simulink model "Frequency_Recovery_Closed_Loop"  (Simulink 8.6)
settings: Solver=FixedStepDiscrete  StartTime=0  StopTime=inf  RelTol=1e-3
InitFcn:
  | % Trainingssequenz
  | trainseq=1/sqrt(2) * ((2*randi([0 1],32,1)-1) + 1i * (2*randi([0 1],32,1)-1));
undefined symbols (not defined in the file): gcbh, rcfiltgaincompat
libraries: commchan3 x1, dspsrcs4 x1, simulink x1, commdigbbndpm3 x1, commrandsrc2 x1, commfilt2 x1
settings Model: Creator=schwall  LastModifiedBy=wunsch
settings DataIOCC: SaveOutput=off  SignalLogging=off  SaveTime=off
settings DebuggingCC: InheritedTsInSrcMsg=none  FcnCallInpInsideContextMsg=UseLocalSettings
settings SFSimCC: SimParseCustomCode=off

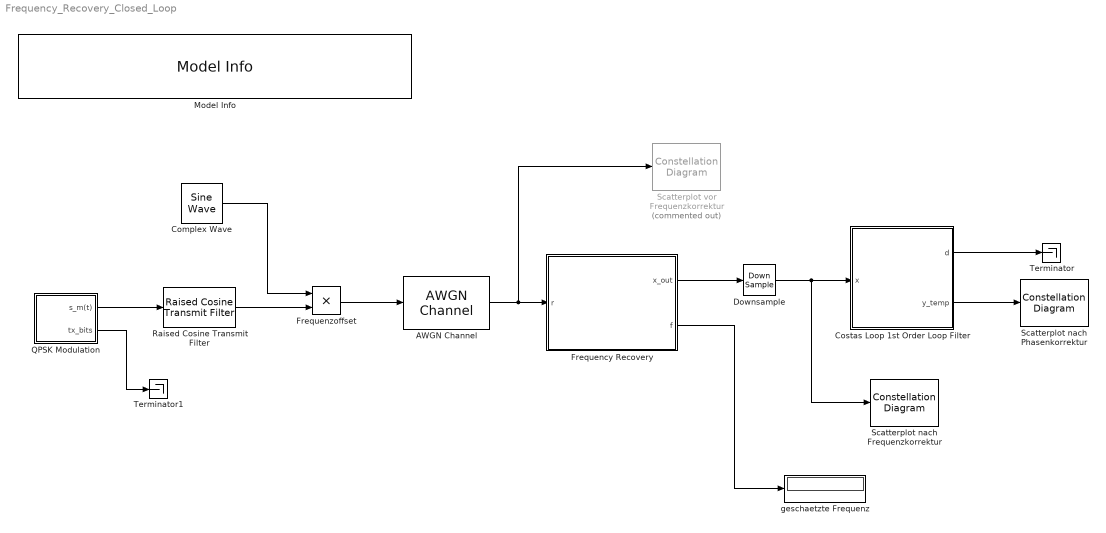
== system Frequency_Recovery_Closed_Loop ==
  AWGN Channel : commchan3/AWGN Channel  InputProcessing=Columns as channels (frame based)  seed=67  noiseMode="Signal to noise ratio  (Es/No)"  EbNodB=12  EsNodB=30  SNRdB=10  bitsPerSym=2  Ps=1/8  Tsym=0.128/128/8  variance=1
  Complex Wave : dspsrcs4/Sine Wave  Amplitude=1  Frequency=0  Phase=0  SampleMode=Discrete  OutComplex=Complex  CompMethod=Trigonometric fcn  TableSize=Speed  SampleTime=0.128/128/8  SamplesPerFrame=1024  ResetState=Restart at time zero  OutputFrames=on  dataType=double  wordLen=16  udDataType=sfix(16)  fracBitsMode=Best precision  numFracBits=15  OutDataTypeStr=double  LastOutDataTypeStr=double
  Costas Loop 1st Order Loop Filter : MATLAB Function  TreatAsAtomicUnit=on
  Downsample : DownSample
  Frequency Recovery : MATLAB Function  TreatAsAtomicUnit=on
  Frequenzoffset : Product  RndMeth=Zero
  Model Info : simulink/Model-Wide Utilities/Model Info  BlockCM=None  Frame=on  DisplayStringWithTags=|  HorizontalTextAlignment=Left  LeftAlignmentValue=0.02  SourceBlockDiagram=Frequency_Recovery_Closed_Loop  TagMaxNumber=20
      | Demo Frequency Recovery Closed Loop
      | Vorlesung Nachrichtentechnik II
      | Institut fuer Nachrichtentechnik (CEL)
  QPSK Modulation : Subsystem
  Raised Cosine Transmit Filter : commfilt2/Raised Cosine Transmit Filter  filtType=Square root  filtSpan=2*(3)  currentFiltSpan=2*(3)  D=3  R=0.35  sampMode=Mute  saveAsFlag=0  N=8  framing=Enforce single-rate processing  InputProcessing=Columns as channels (frame based)  checkGain=Normalized  filterGain=rcfiltgaincompat(gcbh)  checkCoeff=off  variableName=rcTxFilt  launchFVT=off  roundingMode=Floor  overflowMode=off
  Scatterplot nach Frequenzkorrektur : ConstellationDiagram  Tag=ScatterPlot
  Scatterplot nach Phasenkorrektur : ConstellationDiagram  Tag=ScatterPlot
  Scatterplot vor Frequenzkorrektur : ConstellationDiagram  Tag=ScatterPlot  Commented=on
  Terminator : Terminator
  Terminator1 : Terminator
  geschaetzte Frequenz : Display
  wires:
  QPSK Modulation/1(s_m(t)) -> Raised Cosine Transmit Filter/1
  Frequenzoffset/1 -> AWGN Channel/1
  Complex Wave/1 -> Frequenzoffset/1
  Raised Cosine Transmit Filter/1 -> Frequenzoffset/2
  AWGN Channel/1 -> Scatterplot vor Frequenzkorrektur/1, Frequency Recovery/1(r)
  Frequency Recovery/1(x_out) -> Downsample/1
  Frequency Recovery/2(f) -> geschaetzte Frequenz/1
  Costas Loop 1st Order Loop Filter/2(y_temp) -> Scatterplot nach Phasenkorrektur/1
  Downsample/1 -> Scatterplot nach Frequenzkorrektur/1, Costas Loop 1st Order Loop Filter/1(x)
  Costas Loop 1st Order Loop Filter/1(d) -> Terminator/1
  QPSK Modulation/2(tx_bits) -> Terminator1/1

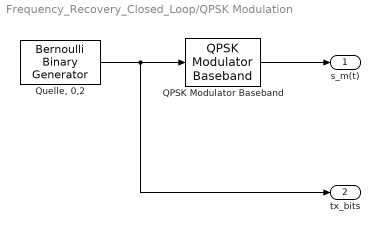
== system Frequency_Recovery_Closed_Loop/QPSK Modulation ==
  QPSK Modulator Baseband : commdigbbndpm3/QPSK Modulator Baseband  InType=Bit  Enc=Gray  Ph=pi/4  outDtype=double  outWordLen=16  outUDDataType=sfix(16)  outFracLenMode=Best precision  outFracLen=15
  "Quelle, 0,2" : commrandsrc2/Bernoulli Binary Generator  P=0.5  seed=61  Ts=1/1000/2  frameBased=on  sampPerFrame=256  orient=off  outDataType=double
  s_m(t) : Outport
  tx_bits : Outport  Port=2
  wires:
  "Quelle, 0,2"/1 -> QPSK Modulator Baseband/1, tx_bits/1
  QPSK Modulator Baseband/1 -> s_m(t)/1

== matlab function Frequency Recovery ==
  data: x_out output double; r input double; f output double
function [x_out,f]  = recovery(r)
%#codegen

%%%%%%%%%%%%%%%%%%%%%%%%%%%%%%%%%%%%%%%%%%%%%%%%%%%%%%%%%%%%%%%%%%%%%%%%%%%
% Initalisierung
%%%%%%%%%%%%%%%%%%%%%%%%%%%%%%%%%%%%%%%%%%%%%%%%%%%%%%%%%%%%%%%%%%%%%%%%%%%

% Impulsantwort Matched Filter
g_mf = [-0.00899923276653125,-0.00862010031857740,-0.00522380865789863,0.00100721609395230,0.00905626800252464,0.0171605778586790,0.0231027321668600,0.0246690244769097,0.0201947243108860,0.00908564037698491,-0.00780385491973082,-0.0280398387740470,-0.0477877316963890,-0.0623056364195982,-0.0666918594078338,-0.0567682669013122,-0.0299425306660226,0.0141173785993224,0.0731400166589809,0.142329093949593,0.214880423378019,0.282872674533704,0.338395135492808,0.374726714857473,0.387365059213122,0.374726714857473,0.338395135492808,0.282872674533704,0.214880423378019,0.142329093949593,0.0731400166589809,0.0141173785993224,-0.0299425306660226,-0.0567682669013122,-0.0666918594078338,-0.0623056364195982,-0.0477877316963890,-0.0280398387740470,-0.00780385491973082,0.00908564037698491,0.0201947243108860,0.0246690244769097,0.0231027321668600,0.0171605778586790,0.00905626800252464,0.00100721609395230,-0.00522380865789863,-0.00862010031857740,-0.00899923276653125];
% Derivative Matched Filter
T = 1;
k = ceil(-length(g_mf)/2):floor(length(g_mf)/2);
g_dmf = 2*pi*T*k.*g_mf;

% Ausgabe initialisieren
x_out = complex(zeros(length(r)/4,1));
f = 0;

% Schrittweite
gamma = 0.01;

% temp. Variable: Speicherinhalt x-Zweig
persistent x_buf
if isempty(x_buf)
    x_buf = complex(zeros(length(g_mf)-1,1));
end

persistent x_1
if isempty(x_1)
    x_1 = complex(0);
end

% temp. Variable: Speicherinhalt y-Zweig
persistent y_buf
if isempty(y_buf)
    y_buf = complex(zeros(length(g_dmf)-1,1));
end

persistent y_1
if isempty(y_1)
    y_1 = complex(0);
end

% Frequenz
persistent nu
if isempty(nu)
    nu = 0;
end

% Phaseninkrement
persistent phi
if isempty(phi)
    phi = 0;
end

% temp. Zaehlervariable
cnt=1;

%%%%%%%%%%%%%%%%%%%%%%%%%%%%%%%%%%%%%%%%%%%%%%%%%%%%%%%%%%%%%%%%%%%%%%%%%%%
% Phasenkorrektur
%%%%%%%%%%%%%%%%%%%%%%%%%%%%%%%%%%%%%%%%%%%%%%%%%%%%%%%%%%%%%%%%%%%%%%%%%%%

for ii=1:length(r)
    
    % Korrektur des Eingangswertes
    r(ii) = r(ii) * exp(1i*(-phi));
    
    % neues Phaseninkrement berechnen
    phi = phi + 2*pi*nu/8000;
    
    % Filteroperationen, MF+DMF
    [x,x_buf] = filter(g_mf, 1,r(ii),x_buf);
    [y,y_buf] = filter(g_dmf,1,r(ii),y_buf);
    
      
    % Downsample by 8
    if (mod(ii,8) == 1)
        
        % Fehler berechnen
        e = 0.5*imag(x_1*conj(y_1)) + 0.5*imag(x*conj(y)); 
        
        % Frequenzoffset berechnen
        nu= nu + gamma*e;     
        
        % nur zur Visualisierung
        f=f+nu;
    end
    
    % Downsample by 4
    if (mod(ii,4) == 1)
        
        x_1 = x;
        y_1 = y;
        
        % Ausgabe, Faktor 2 ueberabgetastet!
        x_out(cnt) = x;
        cnt=cnt+1;
    end    
   
end

% nur zur Visualisierung
f=f/length(r)*8;

== matlab function Costas Loop 1st Order Loop Filter ==
  data: x input double; d output double; y_temp output double
function [d,y_temp] = recovery(x)
%#codegen

%%%%%%%%%%%%%%%%%%%%%%%%%%%%%%%%%%%%%%%%%%%%%%%%%%%%%%%%%%%%%%%%%%%%%%%%%%%
% Initalisierung
%%%%%%%%%%%%%%%%%%%%%%%%%%%%%%%%%%%%%%%%%%%%%%%%%%%%%%%%%%%%%%%%%%%%%%%%%%%

gamma       = 0.5;                          % Schrittweite

persistent phi
if isempty(phi)
    phi = 0;
end

d = complex(zeros(length(x),1));            % Ausgabevektor

y_temp=complex(zeros(length(x),1));         % nur fuer Visualisierungszwecke

%%%%%%%%%%%%%%%%%%%%%%%%%%%%%%%%%%%%%%%%%%%%%%%%%%%%%%%%%%%%%%%%%%%%%%%%%%%
% Phasenkorrektur
%%%%%%%%%%%%%%%%%%%%%%%%%%%%%%%%%%%%%%%%%%%%%%%%%%%%%%%%%%%%%%%%%%%%%%%%%%%

for ii=1:length(x)
    
    
    % Korrektur des Eingangswertes
    y = x(ii) * exp(1i*(-phi));
    
    % nur fuer Visualisierungszwecke
    y_temp(ii) = y;
    
    % Detektor
    d(ii) = detector(y);
    
      
    % Bestimmung des Phasenkorrekturwertes
    phi = phi + gamma * imag( conj(d(ii)) * y );
    
    
end

end


%%%%%%%%%%%%%%%%%%%%%%%%%%%%%%%%%%%%%%%%%%%%%%%%%%%%%%%%%%%%%%%%%%%%%%%%%%%
% QPSK-Detektor
%%%%%%%%%%%%%%%%%%%%%%%%%%%%%%%%%%%%%%%%%%%%%%%%%%%%%%%%%%%%%%%%%%%%%%%%%%%
function d = detector(y)

    % Ueberpruefung der Entscheidungsgebiete
    if     (real(y) >= 0 && imag(y) >= 0)
        d = 1/sqrt(2) * (1+1i);
    elseif (real(y)  < 0 && imag(y) >= 0)
        d = 1/sqrt(2) * (-1+1i);
    elseif (real(y)  < 0 && imag(y)  < 0)
        d = 1/sqrt(2) * (-1-1i);
    else
        d = 1/sqrt(2) * (1-1i);
    end
end
